simulink model "scdsaturationDFcl"  (Simulink 7.6)
settings: Solver=ode45  StartTime=0.0  StopTime=10.0  RelTol=1e-3
settings Model: Creator=The MathWorks Inc.
settings DebuggingCC: SolverPrmCheckMsg=none  StrictBusMsg=Warning

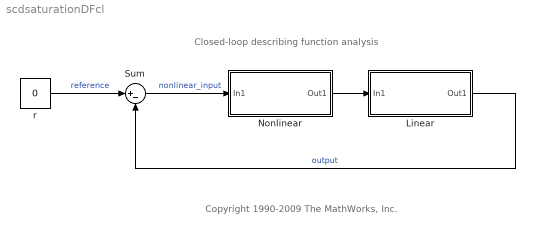
== system scdsaturationDFcl ==
  note: Closed-loop describing function analysis
  note: Copyright 1990-2009 The MathWorks, Inc.
  Linear : Subsystem
  Nonlinear : Subsystem
  Sum : Sum  Inputs=|+-
  r : Constant  Value=0
  wires:
  Sum/1 -> Nonlinear/1(In1)  "nonlinear_input"
  Nonlinear/1(Out1) -> Linear/1(In1)
  Linear/1(Out1) -> Sum/2  "output"
  r/1 -> Sum/1  "reference"

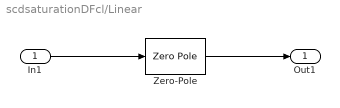
== system scdsaturationDFcl/Linear ==
  In1 : Inport
  Zero-Pole : ZeroPole  Zeros=[]  Poles=[0 -1 -10]
  Out1 : Outport
  wires:
  In1/1 -> Zero-Pole/1
  Zero-Pole/1 -> Out1/1

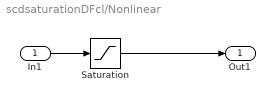
== system scdsaturationDFcl/Nonlinear ==
  In1 : Inport
  Saturation : Saturate
  Out1 : Outport
  wires:
  In1/1 -> Saturation/1
  Saturation/1 -> Out1/1
